simulink model "simumodel"  (Simulink 8.0)
settings: Solver=ode4  StartTime=0.0  StopTime=stop_time  FixedStep=step_time  RelTol=1e-3
values from neighbouring files (symbols this model uses):
  C_Den = [0 1]    [main_1.m]
  C_Num = [1]    [main_1.m]
  Exp_Lamda = 7.9    [main_1.m]
  mean_wind = 15    [main_1.m]
  R = 38.5    [main_1.m]    (also in test.m)
settings Model: Creator=acer  LastModifiedBy=dujiexian
settings DataIOCC: SignalLoggingSaveFormat=ModelDataLogs
settings OptimizationCC: InitFltsAndDblsToZero=on
settings DebuggingCC: SaveWithParameterizedLinksMsg=none  SignalResolutionControl=TryResolveAllWithWarning  MultiTaskDSMMsg=warning  MultiTaskCondExecSysMsg=none  FcnCallInpInsideContextMsg=UseLocalSettings  StrictBusMsg=Warning
settings RTWCC: IncludeERTFirstTime=on
settings GRTTargetCC: TargetFcnLib=ansi_tfl_tmw.mat  CombineOutputUpdateFcns=off  GRTInterface=on

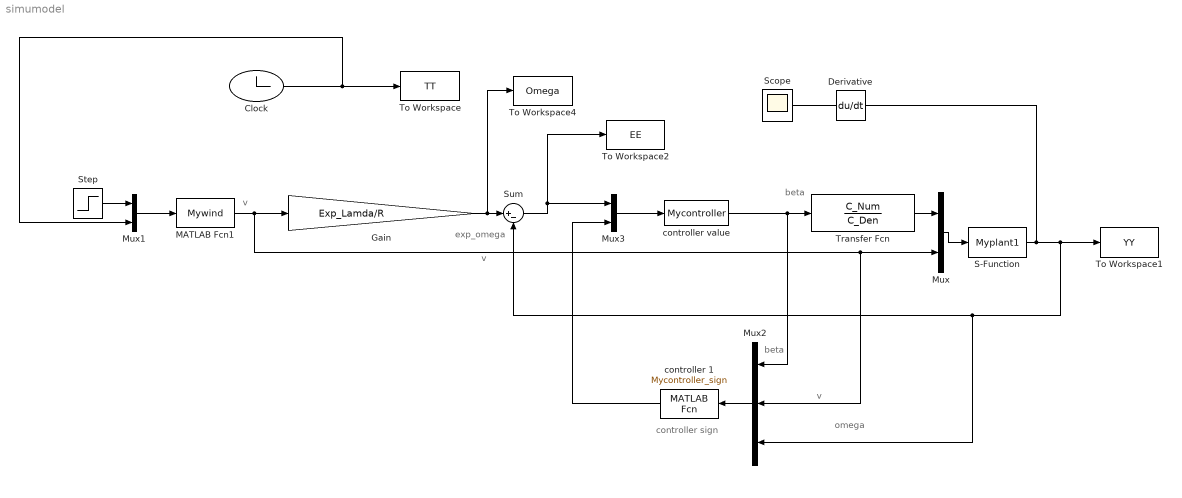
== system simumodel ==
  note: beta
  note: v
  note: v
  note: exp_omega
  note: beta
  note: v
  note: omega
  note: controller sign
  Clock : Clock
  Derivative : Derivative
  Gain : Gain  Gain=Exp_Lamda/R
  MATLAB Fcn1 : MATLABFcn  MATLABFcn=Mywind
  Mux : Mux  Inputs=2
  Mux1 : Mux  Inputs=2
  Mux2 : Mux  Inputs=3
  Mux3 : Mux  Inputs=2
  S-Function : S-Function  FunctionName=Myplant1  EnableBusSupport=off
  Scope : Scope
  Step : Step  Time=0  After=mean_wind  SampleTime=0
  Sum : Sum  Inputs=|+-
  To Workspace : ToWorkspace  VariableName=TT  SampleTime=-1
  To Workspace1 : ToWorkspace  VariableName=YY  SampleTime=-1
  To Workspace2 : ToWorkspace  VariableName=EE  SampleTime=-1
  To Workspace4 : ToWorkspace  VariableName=Omega  SampleTime=-1
  Transfer Fcn : TransferFcn  Numerator=C_Num  Denominator=C_Den
  controller 1 : MATLABFcn  MATLABFcn=Mycontroller_sign
  "controller value " : MATLABFcn  MATLABFcn=Mycontroller  OutputDimensions=1
  wires:
  Clock/1 -> To Workspace/1, Mux1/2
  MATLAB Fcn1/1 -> Gain/1, Mux/2, Mux2/2
  Sum/1 -> To Workspace2/1, Mux3/1
  Mux/1 -> S-Function/1
  S-Function/1 -> To Workspace1/1, Sum/2, Mux2/3, Derivative/1
  Transfer Fcn/1 -> Mux/1
  Derivative/1 -> Scope/1
  Step/1 -> Mux1/1
  Mux1/1 -> MATLAB Fcn1/1
  "controller value "/1 -> Transfer Fcn/1, Mux2/1
  Mux2/1 -> controller 1/1
  Mux3/1 -> "controller value "/1
  controller 1/1 -> Mux3/2
  Gain/1 -> To Workspace4/1, Sum/1
